simulink model "Vehicle_Model"  (R2018b)
settings: Solver=VariableStepAuto  StartTime=0.0  StopTime=60  FixedStep=0.00000000000000000000000000000000000000001  RelTol=1e-3
undefined symbols (not defined in the file or in its folder): Chassis8_Initial, Initial
(part 1 of 3)
settings Model: Creator=Foster  LastModifiedBy=Will

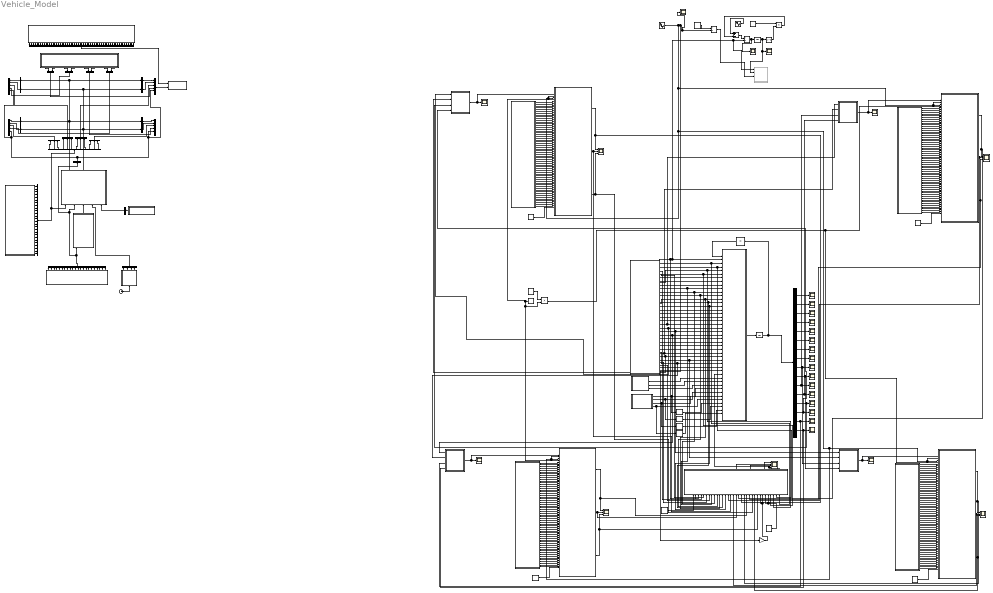
== system Vehicle_Model ==
  note: F=ma for Car in x
  note: Track Radius
  note: Track Curvature
  note: Tyre Model
  note: Rear Right
  note: Rear Left
  note: Front Right
  note: Front Left
  note: 8 DOF Chassis Ride Model
  note: Tyre Model
  note: Tyre Model
  note: Tyre Model
  Bus Creator : BusCreator  Inputs=22
  Bus Creator1 : BusCreator  Inputs=4
  Bus Creator{9..12} (4 alike) : BusCreator  Inputs=3
  Bus Creator{13..16} (4 alike) : BusCreator  Inputs=2
  Bus Creator{2..5} (4 alike) : BusCreator  Inputs=6
  Bus Creator6 : BusCreator  Inputs=59
  Bus Creator7 : BusCreator  Inputs=26
  Bus Creator8 : BusCreator  Inputs=1
  Bus Selector : BusSelector  OutputSignals=x_WFR
  Bus Selector1 : BusSelector  OutputSignals=x_WFL
  Bus Selector2 : BusSelector  OutputSignals=x_WRL
  Bus Selector3 : BusSelector  OutputSignals=x_WRR
  Bus Selector4 : BusSelector  OutputSignals=xdot_WFL
  Bus Selector5 : BusSelector  OutputSignals=xdot_WRL
  Bus Selector6 : BusSelector  OutputSignals=xdot_WFR
  Bus Selector7 : BusSelector  OutputSignals=xdot_WRR
  Bus Selector8 : BusSelector  OutputSignals=mu_scaling
  Bus Selector9 : BusSelector  OutputSignals=k_TRL,c_TRL,gamma_RL,k_TFL,c_TFL,gamma_FL,k_TFR,c_TFR,gamma_FR,k_TRR,c_TRR,gamma_RR
  Chassis Vertical 8DOF : Subsystem
  Clock : Clock
  Constant : Constant  Value=0.0175
  Constant{1..4} (4 alike) : Constant  Value=0.5
  Constant5 : Constant  Value=-1
  Constant6 : Constant
  Constant7 : Constant  Value=9.81
  Constant8 : Constant  Value=0
  Demux : Demux  Outputs=16
  Derivative{,1..3} (4 alike) : Derivative
  Divide : Product  Inputs=*/
  Divide1 : Product  Inputs=*/
  Drag Coefficient : Constant  Value=5
  Force_FL : Scope
  Force_FR : Scope
  Force_RL : Scope
  Force_RR : Scope
  Gain : Gain  Gain=50
  IC : InitialCondition  Value=Initial
  Integrator : Integrator
  Integrator1 : Integrator
  MATLAB Function : MATLAB Function  TreatAsAtomicUnit=on
  MATLAB Function1 : MATLAB Function  TreatAsAtomicUnit=on
  MATLAB Function10 : MATLAB Function  TreatAsAtomicUnit=on
  MATLAB Function11 : MATLAB Function  TreatAsAtomicUnit=on
  MATLAB Function12 : MATLAB Function  TreatAsAtomicUnit=on
  MATLAB Function13 : MATLAB Function  TreatAsAtomicUnit=on
  MATLAB Function14 : MATLAB Function  TreatAsAtomicUnit=on
  MATLAB Function15 : MATLAB Function  TreatAsAtomicUnit=on
  MATLAB Function16 : MATLAB Function  Commented=on  TreatAsAtomicUnit=on
  MATLAB Function17 : MATLAB Function  TreatAsAtomicUnit=on
  MATLAB Function18 : MATLAB Function  TreatAsAtomicUnit=on
  MATLAB Function19 : MATLAB Function  TreatAsAtomicUnit=on
  MATLAB Function2 : MATLAB Function  TreatAsAtomicUnit=on
  MATLAB Function20 : MATLAB Function  TreatAsAtomicUnit=on
  MATLAB Function21 : MATLAB Function  TreatAsAtomicUnit=on
  MATLAB Function22 : MATLAB Function  TreatAsAtomicUnit=on
  MATLAB Function23 : MATLAB Function  TreatAsAtomicUnit=on
  MATLAB Function3 : MATLAB Function  TreatAsAtomicUnit=on
  MATLAB Function4 : MATLAB Function  TreatAsAtomicUnit=on
  MATLAB Function5 : MATLAB Function  TreatAsAtomicUnit=on
  MATLAB Function6 : MATLAB Function  TreatAsAtomicUnit=on
  MATLAB Function7 : MATLAB Function  TreatAsAtomicUnit=on
  MATLAB Function8 : MATLAB Function  TreatAsAtomicUnit=on
  MATLAB Function9 : MATLAB Function  TreatAsAtomicUnit=on
  Minus : Sum  Inputs=+-
  Multiply : Product
  Multiply1 : Product
  Scope : Scope
  Scope{1..4} (4 alike) : Scope  NumInputPorts=3
  Scope5 : Scope  NumInputPorts=4
  Sine Wave : Sin  Amplitude=500  Bias=500  Frequency=0.5  SampleTime=0
  Square : Math  Operator=square  SaturateOnIntegerOverflow=on
  Subsystem : Subsystem
  Subsystem1 : Subsystem
  Track Curvature : Sin  Amplitude=0.01  Frequency=0.1  SampleTime=0
  a_x : Scope
  v_x : Scope
  x_WFL : Scope
  x_WFR : Scope
  x_WRL : Scope
  x_WRR : Scope
  x_thetaCF : Scope
  x_thetaCR : Scope
  xdot_WFL : Scope
  xdot_WFR : Scope
  xdot_WRL : Scope
  xdot_WRR : Scope
  xdot_thetaCF : Scope
  xdot_thetaCR : Scope
  y_thetaC : Scope
  ydot_thetaC : Scope
  z_C : Scope
  zdot_C : Scope
  wires:
  MATLAB Function1/1(m_C) -> MATLAB Function/2(m_C), MATLAB Function16/1(m_C), Divide1/2, MATLAB Function18/2(m_C)
  MATLAB Function1/4(m_WFR) -> MATLAB Function18/33(m_WFR), MATLAB Function/3(m_WFR)
  MATLAB Function1/5(m_WFL) -> MATLAB Function/4(m_WFL), MATLAB Function18/32(m_WFL)
  MATLAB Function1/6(m_WRR) -> MATLAB Function/5(m_WRR), MATLAB Function18/31(m_WRR)
  MATLAB Function1/7(m_WRL) -> MATLAB Function/6(m_WRL), MATLAB Function18/30(m_WRL)
  MATLAB Function1/8(I_Cy) -> MATLAB Function/7(I_Cy)
  MATLAB Function1/9(I_CFx) -> MATLAB Function/8(I_CFx)
  MATLAB Function1/10(I_CRx) -> MATLAB Function/9(I_CRx)
  MATLAB Function1/11(a) -> MATLAB Function/10(a), MATLAB Function18/8(a)
  MATLAB Function1/12(b) -> MATLAB Function18/9(b), MATLAB Function/11(b)
  MATLAB Function1/13(d_F) -> MATLAB Function18/10(d_F), MATLAB Function/12(d_F)
  MATLAB Function1/15(d_R) -> MATLAB Function/14(d_R), MATLAB Function18/12(d_R)
  MATLAB Function1/16(e_R) -> MATLAB Function/15(e_R), MATLAB Function18/13(e_R)
  MATLAB Function1/17(k_SFR) -> MATLAB Function/16(k_SFR)
  MATLAB Function1/18(k_SFL) -> MATLAB Function/17(k_SFL)
  MATLAB Function1/19(k_SRR) -> MATLAB Function/18(k_SRR)
  MATLAB Function1/20(k_SRL) -> MATLAB Function/19(k_SRL)
  MATLAB Function1/21(k_TFR) -> MATLAB Function4/1(k), MATLAB Function/20(k_TFR)
  MATLAB Function1/22(k_TFL) -> MATLAB Function7/1(k), MATLAB Function/21(k_TFL)
  MATLAB Function1/23(k_TRR) -> MATLAB Function6/1(k), MATLAB Function/22(k_TRR)
  MATLAB Function1/24(k_TRL) -> MATLAB Function5/1(k), MATLAB Function/23(k_TRL)
  MATLAB Function1/25(c_SFR) -> MATLAB Function/24(c_SFR)
  MATLAB Function1/26(c_SFL) -> MATLAB Function/25(c_SFL)
  MATLAB Function1/27(c_SRR) -> MATLAB Function/26(c_SRR)
  MATLAB Function1/28(c_SRL) -> MATLAB Function/27(c_SRL)
  MATLAB Function1/29(c_TFR) -> MATLAB Function4/2(c), MATLAB Function/28(c_TFR)
  MATLAB Function1/30(c_TFL) -> MATLAB Function7/2(c), MATLAB Function/29(c_TFL)
  MATLAB Function1/31(c_TRR) -> MATLAB Function6/2(c), MATLAB Function/30(c_TRR)
  MATLAB Function1/32(c_TRL) -> MATLAB Function5/2(c), MATLAB Function/31(c_TRL)
  MATLAB Function1/33(k_C) -> MATLAB Function/32(k_C)
  MATLAB Function1/34(c_C) -> MATLAB Function/33(c_C)
  MATLAB Function3/1(y_FR) -> Derivative/1, MATLAB Function/38(y_FR)
  MATLAB Function3/2(y_FL) -> Derivative1/1, MATLAB Function/39(y_FL)
  MATLAB Function3/3(y_RR) -> MATLAB Function/40(y_RR), Derivative2/1
  Derivative/1 -> MATLAB Function/42(ydot_FR)
  Derivative1/1 -> MATLAB Function/43(ydot_FL)
  Derivative2/1 -> MATLAB Function/44(ydot_RR)
  MATLAB Function/1(Z) -> Integrator/1
  Integrator/1 -> IC/1, Demux/1
  Demux/16 -> MATLAB Function5/4(xdot), xdot_WRL/1
  Demux/15 -> MATLAB Function5/3(x), x_WRL/1
  Demux/14 -> MATLAB Function7/4(xdot), xdot_WFL/1
  Demux/13 -> MATLAB Function7/3(x), x_WFL/1
  Demux/12 -> MATLAB Function4/4(xdot), xdot_WFR/1
  Demux/11 -> MATLAB Function4/3(x), x_WFR/1
  Demux/10 -> MATLAB Function6/4(xdot), xdot_WRR/1
  Demux/9 -> MATLAB Function6/3(x), x_WRR/1
  Demux/8 -> xdot_thetaCR/1
  Demux/7 -> x_thetaCR/1
  Demux/6 -> xdot_thetaCF/1
  Demux/5 -> x_thetaCF/1
  Demux/4 -> ydot_thetaC/1
  Demux/3 -> y_thetaC/1
  Demux/2 -> zdot_C/1
  Demux/1 -> z_C/1
  MATLAB Function7/1(F_z) -> MATLAB Function8/1(Fz), Force_FL/1
  MATLAB Function4/1(F_z) -> MATLAB Function14/1(Fz), Force_FR/1
  MATLAB Function6/1(F_z) -> MATLAB Function12/1(Fz), Force_RR/1
  MATLAB Function5/1(F_z) -> MATLAB Function10/1(Fz), Force_RL/1
  Derivative3/1 -> MATLAB Function/45(ydot_RL)
  MATLAB Function9/1(Fzo) -> MATLAB Function8/5(Fzo)
  MATLAB Function9/2(Ro) -> MATLAB Function8/6(Ro)
  MATLAB Function9/3(q_Bz1) -> MATLAB Function8/7(q_Bz1)
  MATLAB Function9/5(q_Bz3) -> MATLAB Function8/9(q_Bz3)
  MATLAB Function9/4(q_Bz2) -> MATLAB Function8/8(q_Bz2)
  MATLAB Function9/6(q_Bz4) -> MATLAB Function8/10(q_Bz4)
  MATLAB Function9/7(q_Bz5) -> MATLAB Function8/11(q_Bz5)
  MATLAB Function9/10(q_Cz1) -> MATLAB Function8/14(q_Cz1)
  MATLAB Function9/9(q_Bz10) -> MATLAB Function8/13(q_Bz10)
  MATLAB Function9/8(q_Bz9) -> MATLAB Function8/12(q_Bz9)
  MATLAB Function9/11(q_Dz1) -> MATLAB Function8/15(q_Dz1)
  MATLAB Function9/12(q_Dz2) -> MATLAB Function8/16(q_Dz2)
  MATLAB Function9/14(q_Dz4) -> MATLAB Function8/18(q_Dz4)
  MATLAB Function9/13(q_Dz3) -> MATLAB Function8/17(q_Dz3)
  MATLAB Function9/15(q_Dz6) -> MATLAB Function8/19(q_Dz6)
  MATLAB Function9/17(q_Dz8) -> MATLAB Function8/21(q_Dz8)
  MATLAB Function9/18(q_Dz9) -> MATLAB Function8/22(q_Dz9)
  MATLAB Function9/20(q_Ez2) -> MATLAB Function8/24(q_Ez2)
  MATLAB Function9/21(q_Ez3) -> MATLAB Function8/25(q_Ez3)
  MATLAB Function9/19(q_Ez1) -> MATLAB Function8/23(q_Ez1)
  MATLAB Function9/22(q_Ez4) -> MATLAB Function8/26(q_Ez4)
  MATLAB Function9/23(q_Ez5) -> MATLAB Function8/27(q_Ez5)
  MATLAB Function9/25(q_Hz2) -> MATLAB Function8/29(q_Hz2)
  MATLAB Function9/24(q_Hz1) -> MATLAB Function8/28(q_Hz1)
  MATLAB Function9/26(q_Hz3) -> MATLAB Function8/30(q_Hz3)
  MATLAB Function9/27(q_Hz4) -> MATLAB Function8/31(q_Hz4)
  MATLAB Function9/28(p_Cy1) -> MATLAB Function8/32(p_Cy1)
  MATLAB Function9/29(p_Dy1) -> MATLAB Function8/33(p_Dy1)
  MATLAB Function9/30(p_Dy2) -> MATLAB Function8/34(p_Dy2)
  MATLAB Function9/31(p_Dy3) -> MATLAB Function8/35(p_Dy3)
  MATLAB Function9/32(p_Ey1) -> MATLAB Function8/36(p_Ey1)
  MATLAB Function9/34(p_Ey3) -> MATLAB Function8/38(p_Ey3)
  MATLAB Function9/33(p_Ey2) -> MATLAB Function8/37(p_Ey2)
  MATLAB Function9/35(p_Ey4) -> MATLAB Function8/39(p_Ey4)
  MATLAB Function9/36(p_Ky1) -> MATLAB Function8/40(p_Ky1)
  MATLAB Function9/37(p_Ky2) -> MATLAB Function8/41(p_Ky2)
  MATLAB Function9/38(p_Ky3) -> MATLAB Function8/42(p_Ky3)
  MATLAB Function9/40(p_Hy2) -> MATLAB Function8/44(p_Hy2)
  MATLAB Function9/39(p_Hy1) -> MATLAB Function8/43(p_Hy1)
  MATLAB Function9/41(p_Hy3) -> MATLAB Function8/45(p_Hy3)
  MATLAB Function9/42(p_Vy1) -> MATLAB Function8/46(p_Vy1)
  MATLAB Function9/44(p_Vy3) -> MATLAB Function8/48(p_Vy3)
  MATLAB Function9/43(p_Vy2) -> MATLAB Function8/47(p_Vy2)
  MATLAB Function9/46(p_Cx1) -> MATLAB Function8/50(p_Cx1)
  MATLAB Function9/45(p_Vy4) -> MATLAB Function8/49(p_Vy4)
  MATLAB Function9/47(p_Dx1) -> MATLAB Function8/51(p_Dx1)
  MATLAB Function9/48(p_Dx2) -> MATLAB Function8/52(p_Dx2)
  MATLAB Function9/49(p_Ex1) -> MATLAB Function8/53(p_Ex1)
  MATLAB Function9/50(p_Ex2) -> MATLAB Function8/54(p_Ex2)
  MATLAB Function9/51(p_Ex3) -> MATLAB Function8/55(p_Ex3)
  MATLAB Function9/52(p_Ex4) -> MATLAB Function8/56(p_Ex4)
  MATLAB Function9/53(p_Kx1) -> MATLAB Function8/57(p_Kx1)
  MATLAB Function9/54(p_Kx2) -> MATLAB Function8/58(p_Kx2)
  MATLAB Function9/55(p_Kx3) -> MATLAB Function8/59(p_Kx3)
  MATLAB Function9/56(p_Hx1) -> MATLAB Function8/60(p_Hx1)
  MATLAB Function9/57(p_Hx2) -> MATLAB Function8/61(p_Hx2)
  MATLAB Function9/58(p_Vx1) -> MATLAB Function8/62(p_Vx1)
  MATLAB Function9/59(p_Vx2) -> MATLAB Function8/63(p_Vx2)
  Constant1/1 -> MATLAB Function8/64(car_mu_scaling)
  MATLAB Function9/16(q_Dz7) -> MATLAB Function8/20(q_Dz7)
  MATLAB Function8/1(Fxo) -> MATLAB Function18/19(F_xFL), Scope1/1
  MATLAB Function8/2(Fyo) -> MATLAB Function18/15(F_yFL), Scope1/2
  MATLAB Function8/3(Mzo) -> MATLAB Function18/23(M_zFL), Scope1/3
  MATLAB Function10/2(Fyo) -> MATLAB Function18/17(F_yRL), Scope2/2
  MATLAB Function11/56(p_Hx1) -> MATLAB Function10/60(p_Hx1)
  MATLAB Function11/40(p_Hy2) -> MATLAB Function10/44(p_Hy2)
  MATLAB Function11/9(q_Bz10) -> MATLAB Function10/13(q_Bz10)
  MATLAB Function11/26(q_Hz3) -> MATLAB Function10/30(q_Hz3)
  MATLAB Function11/52(p_Ex4) -> MATLAB Function10/56(p_Ex4)
  MATLAB Function11/35(p_Ey4) -> MATLAB Function10/39(p_Ey4)
  MATLAB Function11/5(q_Bz3) -> MATLAB Function10/9(q_Bz3)
  MATLAB Function11/7(q_Bz5) -> MATLAB Function10/11(q_Bz5)
  MATLAB Function11/21(q_Ez3) -> MATLAB Function10/25(q_Ez3)
  MATLAB Function11/38(p_Ky3) -> MATLAB Function10/42(p_Ky3)
  MATLAB Function11/14(q_Dz4) -> MATLAB Function10/18(q_Dz4)
  MATLAB Function11/51(p_Ex3) -> MATLAB Function10/55(p_Ex3)
  MATLAB Function11/45(p_Vy4) -> MATLAB Function10/49(p_Vy4)
  MATLAB Function11/18(q_Dz9) -> MATLAB Function10/22(q_Dz9)
  MATLAB Function11/37(p_Ky2) -> MATLAB Function10/41(p_Ky2)
  MATLAB Function11/39(p_Hy1) -> MATLAB Function10/43(p_Hy1)
  MATLAB Function11/55(p_Kx3) -> MATLAB Function10/59(p_Kx3)
  MATLAB Function11/59(p_Vx2) -> MATLAB Function10/63(p_Vx2)
  MATLAB Function11/4(q_Bz2) -> MATLAB Function10/8(q_Bz2)
  MATLAB Function11/24(q_Hz1) -> MATLAB Function10/28(q_Hz1)
  MATLAB Function11/15(q_Dz6) -> MATLAB Function10/19(q_Dz6)
  MATLAB Function11/41(p_Hy3) -> MATLAB Function10/45(p_Hy3)
  MATLAB Function10/3(Mzo) -> MATLAB Function18/25(M_zRL), Scope2/3
  MATLAB Function11/50(p_Ex2) -> MATLAB Function10/54(p_Ex2)
  MATLAB Function10/1(Fxo) -> MATLAB Function18/21(F_xRL), Scope2/1
  MATLAB Function11/49(p_Ex1) -> MATLAB Function10/53(p_Ex1)
  MATLAB Function11/46(p_Cx1) -> MATLAB Function10/50(p_Cx1)
  MATLAB Function11/58(p_Vx1) -> MATLAB Function10/62(p_Vx1)
  MATLAB Function11/47(p_Dx1) -> MATLAB Function10/51(p_Dx1)
  MATLAB Function11/48(p_Dx2) -> MATLAB Function10/52(p_Dx2)
  MATLAB Function11/2(Ro) -> MATLAB Function10/6(Ro)
  MATLAB Function11/57(p_Hx2) -> MATLAB Function10/61(p_Hx2)
  MATLAB Function11/54(p_Kx2) -> MATLAB Function10/58(p_Kx2)
  MATLAB Function11/16(q_Dz7) -> MATLAB Function10/20(q_Dz7)
  MATLAB Function11/53(p_Kx1) -> MATLAB Function10/57(p_Kx1)
  Constant2/1 -> MATLAB Function10/64(car_mu_scaling)
  MATLAB Function11/12(q_Dz2) -> MATLAB Function10/16(q_Dz2)
  MATLAB Function11/8(q_Bz9) -> MATLAB Function10/12(q_Bz9)
  MATLAB Function11/19(q_Ez1) -> MATLAB Function10/23(q_Ez1)
  MATLAB Function11/34(p_Ey3) -> MATLAB Function10/38(p_Ey3)
  MATLAB Function11/42(p_Vy1) -> MATLAB Function10/46(p_Vy1)
  MATLAB Function11/1(Fzo) -> MATLAB Function10/5(Fzo)
  MATLAB Function11/20(q_Ez2) -> MATLAB Function10/24(q_Ez2)
  MATLAB Function11/25(q_Hz2) -> MATLAB Function10/29(q_Hz2)
  MATLAB Function11/36(p_Ky1) -> MATLAB Function10/40(p_Ky1)
  MATLAB Function11/32(p_Ey1) -> MATLAB Function10/36(p_Ey1)
  MATLAB Function11/29(p_Dy1) -> MATLAB Function10/33(p_Dy1)
  MATLAB Function11/22(q_Ez4) -> MATLAB Function10/26(q_Ez4)
  MATLAB Function11/31(p_Dy3) -> MATLAB Function10/35(p_Dy3)
  MATLAB Function11/10(q_Cz1) -> MATLAB Function10/14(q_Cz1)
  MATLAB Function11/27(q_Hz4) -> MATLAB Function10/31(q_Hz4)
  MATLAB Function11/23(q_Ez5) -> MATLAB Function10/27(q_Ez5)
  MATLAB Function11/13(q_Dz3) -> MATLAB Function10/17(q_Dz3)
  MATLAB Function11/33(p_Ey2) -> MATLAB Function10/37(p_Ey2)
  MATLAB Function11/43(p_Vy2) -> MATLAB Function10/47(p_Vy2)
  MATLAB Function11/28(p_Cy1) -> MATLAB Function10/32(p_Cy1)
  MATLAB Function11/44(p_Vy3) -> MATLAB Function10/48(p_Vy3)
  MATLAB Function11/3(q_Bz1) -> MATLAB Function10/7(q_Bz1)
  MATLAB Function11/30(p_Dy2) -> MATLAB Function10/34(p_Dy2)
  MATLAB Function11/17(q_Dz8) -> MATLAB Function10/21(q_Dz8)
  MATLAB Function11/6(q_Bz4) -> MATLAB Function10/10(q_Bz4)
  MATLAB Function11/11(q_Dz1) -> MATLAB Function10/15(q_Dz1)
  MATLAB Function13/27(q_Hz4) -> MATLAB Function12/31(q_Hz4)
  MATLAB Function13/18(q_Dz9) -> MATLAB Function12/22(q_Dz9)
  MATLAB Function13/9(q_Bz10) -> MATLAB Function12/13(q_Bz10)
  MATLAB Function13/42(p_Vy1) -> MATLAB Function12/46(p_Vy1)
  MATLAB Function13/45(p_Vy4) -> MATLAB Function12/49(p_Vy4)
  MATLAB Function13/30(p_Dy2) -> MATLAB Function12/34(p_Dy2)
  MATLAB Function13/33(p_Ey2) -> MATLAB Function12/37(p_Ey2)
  MATLAB Function13/37(p_Ky2) -> MATLAB Function12/41(p_Ky2)
  MATLAB Function13/7(q_Bz5) -> MATLAB Function12/11(q_Bz5)
  MATLAB Function13/20(q_Ez2) -> MATLAB Function12/24(q_Ez2)
  MATLAB Function13/52(p_Ex4) -> MATLAB Function12/56(p_Ex4)
  MATLAB Function13/28(p_Cy1) -> MATLAB Function12/32(p_Cy1)
  MATLAB Function13/43(p_Vy2) -> MATLAB Function12/47(p_Vy2)
  MATLAB Function13/22(q_Ez4) -> MATLAB Function12/26(q_Ez4)
  MATLAB Function13/21(q_Ez3) -> MATLAB Function12/25(q_Ez3)
  MATLAB Function13/44(p_Vy3) -> MATLAB Function12/48(p_Vy3)
  MATLAB Function13/31(p_Dy3) -> MATLAB Function12/35(p_Dy3)
  MATLAB Function13/55(p_Kx3) -> MATLAB Function12/59(p_Kx3)
  MATLAB Function13/39(p_Hy1) -> MATLAB Function12/43(p_Hy1)
  MATLAB Function13/11(q_Dz1) -> MATLAB Function12/15(q_Dz1)
  MATLAB Function12/2(Fyo) -> MATLAB Function18/16(F_yRR), Scope3/2
  MATLAB Function13/56(p_Hx1) -> MATLAB Function12/60(p_Hx1)
  MATLAB Function13/5(q_Bz3) -> MATLAB Function12/9(q_Bz3)
  MATLAB Function13/14(q_Dz4) -> MATLAB Function12/18(q_Dz4)
  MATLAB Function13/35(p_Ey4) -> MATLAB Function12/39(p_Ey4)
  MATLAB Function13/13(q_Dz3) -> MATLAB Function12/17(q_Dz3)
  MATLAB Function13/40(p_Hy2) -> MATLAB Function12/44(p_Hy2)
  MATLAB Function13/46(p_Cx1) -> MATLAB Function12/50(p_Cx1)
  MATLAB Function13/19(q_Ez1) -> MATLAB Function12/23(q_Ez1)
  MATLAB Function13/36(p_Ky1) -> MATLAB Function12/40(p_Ky1)
  MATLAB Function13/38(p_Ky3) -> MATLAB Function12/42(p_Ky3)
  MATLAB Function13/59(p_Vx2) -> MATLAB Function12/63(p_Vx2)
  MATLAB Function13/4(q_Bz2) -> MATLAB Function12/8(q_Bz2)
  MATLAB Function13/32(p_Ey1) -> MATLAB Function12/36(p_Ey1)
  MATLAB Function13/12(q_Dz2) -> MATLAB Function12/16(q_Dz2)
  MATLAB Function13/6(q_Bz4) -> MATLAB Function12/10(q_Bz4)
  MATLAB Function13/3(q_Bz1) -> MATLAB Function12/7(q_Bz1)
  MATLAB Function13/15(q_Dz6) -> MATLAB Function12/19(q_Dz6)
  MATLAB Function13/8(q_Bz9) -> MATLAB Function12/12(q_Bz9)
  Constant3/1 -> MATLAB Function12/64(car_mu_scaling)
  MATLAB Function13/10(q_Cz1) -> MATLAB Function12/14(q_Cz1)
  MATLAB Function13/26(q_Hz3) -> MATLAB Function12/30(q_Hz3)
  MATLAB Function12/1(Fxo) -> MATLAB Function18/20(F_xRR), Scope3/1
  MATLAB Function13/1(Fzo) -> MATLAB Function12/5(Fzo)
  MATLAB Function13/34(p_Ey3) -> MATLAB Function12/38(p_Ey3)
  MATLAB Function13/41(p_Hy3) -> MATLAB Function12/45(p_Hy3)
  MATLAB Function13/23(q_Ez5) -> MATLAB Function12/27(q_Ez5)
  MATLAB Function13/51(p_Ex3) -> MATLAB Function12/55(p_Ex3)
  MATLAB Function13/29(p_Dy1) -> MATLAB Function12/33(p_Dy1)
  MATLAB Function13/17(q_Dz8) -> MATLAB Function12/21(q_Dz8)
  MATLAB Function13/25(q_Hz2) -> MATLAB Function12/29(q_Hz2)
  MATLAB Function13/16(q_Dz7) -> MATLAB Function12/20(q_Dz7)
  MATLAB Function13/2(Ro) -> MATLAB Function12/6(Ro)
  MATLAB Function13/48(p_Dx2) -> MATLAB Function12/52(p_Dx2)
  MATLAB Function13/47(p_Dx1) -> MATLAB Function12/51(p_Dx1)
  MATLAB Function13/53(p_Kx1) -> MATLAB Function12/57(p_Kx1)
  MATLAB Function13/54(p_Kx2) -> MATLAB Function12/58(p_Kx2)
  MATLAB Function13/49(p_Ex1) -> MATLAB Function12/53(p_Ex1)
  MATLAB Function13/24(q_Hz1) -> MATLAB Function12/28(q_Hz1)
  MATLAB Function13/57(p_Hx2) -> MATLAB Function12/61(p_Hx2)
  MATLAB Function12/3(Mzo) -> Scope3/3, MATLAB Function18/24(M_zRR)
  MATLAB Function13/58(p_Vx1) -> MATLAB Function12/62(p_Vx1)
  MATLAB Function13/50(p_Ex2) -> MATLAB Function12/54(p_Ex2)
  MATLAB Function15/27(q_Hz4) -> MATLAB Function14/31(q_Hz4)
  MATLAB Function15/18(q_Dz9) -> MATLAB Function14/22(q_Dz9)
  MATLAB Function15/9(q_Bz10) -> MATLAB Function14/13(q_Bz10)
  MATLAB Function15/42(p_Vy1) -> MATLAB Function14/46(p_Vy1)
  MATLAB Function15/45(p_Vy4) -> MATLAB Function14/49(p_Vy4)
  MATLAB Function15/30(p_Dy2) -> MATLAB Function14/34(p_Dy2)
  MATLAB Function15/33(p_Ey2) -> MATLAB Function14/37(p_Ey2)
  MATLAB Function15/37(p_Ky2) -> MATLAB Function14/41(p_Ky2)
  MATLAB Function15/7(q_Bz5) -> MATLAB Function14/11(q_Bz5)
  MATLAB Function15/20(q_Ez2) -> MATLAB Function14/24(q_Ez2)
  MATLAB Function15/52(p_Ex4) -> MATLAB Function14/56(p_Ex4)
  MATLAB Function15/28(p_Cy1) -> MATLAB Function14/32(p_Cy1)
  MATLAB Function15/43(p_Vy2) -> MATLAB Function14/47(p_Vy2)
  MATLAB Function15/22(q_Ez4) -> MATLAB Function14/26(q_Ez4)
  MATLAB Function15/21(q_Ez3) -> MATLAB Function14/25(q_Ez3)
  MATLAB Function15/44(p_Vy3) -> MATLAB Function14/48(p_Vy3)
  MATLAB Function15/31(p_Dy3) -> MATLAB Function14/35(p_Dy3)
  MATLAB Function15/55(p_Kx3) -> MATLAB Function14/59(p_Kx3)
  MATLAB Function15/39(p_Hy1) -> MATLAB Function14/43(p_Hy1)
  MATLAB Function15/11(q_Dz1) -> MATLAB Function14/15(q_Dz1)
  MATLAB Function14/2(Fyo) -> MATLAB Function18/14(F_yFR), Scope4/2
  MATLAB Function15/56(p_Hx1) -> MATLAB Function14/60(p_Hx1)
  MATLAB Function15/5(q_Bz3) -> MATLAB Function14/9(q_Bz3)
  MATLAB Function15/14(q_Dz4) -> MATLAB Function14/18(q_Dz4)
  MATLAB Function15/35(p_Ey4) -> MATLAB Function14/39(p_Ey4)
  MATLAB Function15/13(q_Dz3) -> MATLAB Function14/17(q_Dz3)
  MATLAB Function15/40(p_Hy2) -> MATLAB Function14/44(p_Hy2)
  MATLAB Function15/46(p_Cx1) -> MATLAB Function14/50(p_Cx1)
  MATLAB Function15/19(q_Ez1) -> MATLAB Function14/23(q_Ez1)
  MATLAB Function15/36(p_Ky1) -> MATLAB Function14/40(p_Ky1)
  MATLAB Function15/38(p_Ky3) -> MATLAB Function14/42(p_Ky3)
  MATLAB Function15/59(p_Vx2) -> MATLAB Function14/63(p_Vx2)
  MATLAB Function15/4(q_Bz2) -> MATLAB Function14/8(q_Bz2)
  MATLAB Function15/32(p_Ey1) -> MATLAB Function14/36(p_Ey1)
  MATLAB Function15/12(q_Dz2) -> MATLAB Function14/16(q_Dz2)
  MATLAB Function15/6(q_Bz4) -> MATLAB Function14/10(q_Bz4)
  MATLAB Function15/3(q_Bz1) -> MATLAB Function14/7(q_Bz1)
  MATLAB Function15/15(q_Dz6) -> MATLAB Function14/19(q_Dz6)
  MATLAB Function15/8(q_Bz9) -> MATLAB Function14/12(q_Bz9)
  Constant4/1 -> MATLAB Function14/64(car_mu_scaling)
  MATLAB Function15/10(q_Cz1) -> MATLAB Function14/14(q_Cz1)
  MATLAB Function15/26(q_Hz3) -> MATLAB Function14/30(q_Hz3)
  MATLAB Function14/1(Fxo) -> MATLAB Function18/18(F_xFR), Scope4/1
  MATLAB Function15/1(Fzo) -> MATLAB Function14/5(Fzo)
  MATLAB Function15/34(p_Ey3) -> MATLAB Function14/38(p_Ey3)
  MATLAB Function15/41(p_Hy3) -> MATLAB Function14/45(p_Hy3)
  MATLAB Function15/23(q_Ez5) -> MATLAB Function14/27(q_Ez5)
  MATLAB Function15/51(p_Ex3) -> MATLAB Function14/55(p_Ex3)
  MATLAB Function15/29(p_Dy1) -> MATLAB Function14/33(p_Dy1)
  MATLAB Function15/17(q_Dz8) -> MATLAB Function14/21(q_Dz8)
  MATLAB Function15/25(q_Hz2) -> MATLAB Function14/29(q_Hz2)
  MATLAB Function15/16(q_Dz7) -> MATLAB Function14/20(q_Dz7)
  MATLAB Function15/2(Ro) -> MATLAB Function14/6(Ro)
  MATLAB Function15/48(p_Dx2) -> MATLAB Function14/52(p_Dx2)
  MATLAB Function15/47(p_Dx1) -> MATLAB Function14/51(p_Dx1)
  MATLAB Function15/53(p_Kx1) -> MATLAB Function14/57(p_Kx1)
  MATLAB Function15/54(p_Kx2) -> MATLAB Function14/58(p_Kx2)
  MATLAB Function15/49(p_Ex1) -> MATLAB Function14/53(p_Ex1)
  MATLAB Function15/24(q_Hz1) -> MATLAB Function14/28(q_Hz1)
  MATLAB Function15/57(p_Hx2) -> MATLAB Function14/61(p_Hx2)
  MATLAB Function14/3(Mzo) -> MATLAB Function18/22(M_zFR), Scope4/3
  MATLAB Function15/58(p_Vx1) -> MATLAB Function14/62(p_Vx1)
  MATLAB Function15/50(p_Ex2) -> MATLAB Function14/54(p_Ex2)
  MATLAB Function3/4(y_RL) -> Derivative3/1, MATLAB Function/41(y_RL)
  Constant/1 -> Multiply/2, MATLAB Function10/4(gam), MATLAB Function8/4(gam)
  Constant5/1 -> Multiply/1
  Multiply/1 -> MATLAB Function12/4(gam), MATLAB Function14/4(gam)
  Constant6/1 -> Divide/1
  Divide1/1 -> a_x/1, Integrator1/1
  Integrator1/1 -> MATLAB Function16/2("v_x "), v_x/1, Square/1
  Square/1 -> Multiply1/2
  Drag Coefficient/1 -> Multiply1/1
  Sine Wave/1 -> Minus/1
  Minus/1 -> Divide1/1
  Divide/1 -> MATLAB Function16/3(r)
  Multiply1/1 -> Minus/2
  Track Curvature/1 -> Gain/1, Scope/1, Divide/2, MATLAB Function14/2(kappa), MATLAB Function14/3(alpha), MATLAB Function10/2(kappa), MATLAB Function10/3(alpha), MATLAB Function12/2(kappa), MATLAB Function12/3(alpha), MATLAB Function8/2(kappa), MATLAB Function8/3(alpha)
  MATLAB Function1/3(m_CR) -> MATLAB Function18/5(m_CR)
  MATLAB Function1/2(m_CF) -> MATLAB Function18/4(m_CF)
  Constant7/1 -> MATLAB Function18/1(g)
  MATLAB Function1/35(h_C) -> MATLAB Function18/3(h_C)
  MATLAB Function1/36(h_CF) -> MATLAB Function18/6(h_CF)
  MATLAB Function1/37(h_CR) -> MATLAB Function18/7(h_CR)
  MATLAB Function1/14(e_F) -> MATLAB Function18/11(e_F), MATLAB Function/13(e_F)
  Gain/1 -> MATLAB Function18/27(S_FL), MATLAB Function18/26(S_FR)
  Constant8/1 -> MATLAB Function18/29(S_RL), MATLAB Function18/28(S_RR)
  IC/1 -> MATLAB Function/1(z)
  MATLAB Function18/7(F_z) -> MATLAB Function/34(F_z), Scope5/4
  MATLAB Function2/3(M_xF) -> MATLAB Function/36(M_xF)
  MATLAB Function2/4(M_xR) -> MATLAB Function/37(M_xR)
  MATLAB Function18/6(M_xR) -> Scope5/1
  MATLAB Function18/5(M_xF) -> Scope5/3
  MATLAB Function18/4(M_y) -> Scope5/2
  MATLAB Function2/2(M_y) -> MATLAB Function/35(M_y)
  MATLAB Function17/1(m_C) -> Bus Creator/1
  MATLAB Function17/2(m_CF) -> Bus Creator/2
  MATLAB Function17/3(m_CR) -> Bus Creator/3
  MATLAB Function17/4(m_WFR) -> Bus Creator/4
  MATLAB Function17/5(m_WFL) -> Bus Creator/5
  MATLAB Function17/6(m_WRR) -> Bus Creator/6
  MATLAB Function17/7(m_WRL) -> Bus Creator/7
  MATLAB Function17/8(I_Cy) -> Bus Creator/8
  MATLAB Function17/9(I_CFx) -> Bus Creator/9
  MATLAB Function17/10(I_CRx) -> Bus Creator/10
  MATLAB Function17/11(a) -> Bus Creator/11
  MATLAB Function17/12(b) -> Bus Creator/12
  MATLAB Function17/13(d_F) -> Bus Creator/13
  MATLAB Function17/14(e_F) -> Bus Creator/14
  MATLAB Function17/15(d_R) -> Bus Creator/15
  MATLAB Function17/16(e_R) -> Bus Creator/16
  MATLAB Function17/17(k_C) -> Bus Creator/17
  MATLAB Function17/18(c_C) -> Bus Creator/18
  MATLAB Function17/19(h_C) -> Bus Creator/19
  MATLAB Function17/20(h_CF) -> Bus Creator/20
  MATLAB Function17/21(h_CR) -> Bus Creator/21
  Bus Creator/1 -> Bus Selector8/1, Chassis Vertical 8DOF/2(Car Parameters), Subsystem/1(Car Parameters)
  MATLAB Function19/1(y_FR) -> Bus Creator1/1
  MATLAB Function19/2(y_FL) -> Bus Creator1/2
  MATLAB Function19/3(y_RR) -> Bus Creator1/3
  MATLAB Function19/4(y_RL) -> Bus Creator1/4
  Bus Creator1/1 -> Chassis Vertical 8DOF/4(Base Excitation)
  Clock/1 -> MATLAB Function19/1(t)
  Subsystem/1(Chassis Forces) -> Chassis Vertical 8DOF/3(Chassis Forces)
  Chassis Vertical 8DOF/1(Vertical Displacements) -> Bus Selector1/1, Bus Selector/1, Bus Selector3/1, Bus Selector2/1
  Chassis Vertical 8DOF/2(Vertical Velocities) -> Bus Selector6/1, Bus Selector4/1, Bus Selector7/1, Bus Selector5/1
  Bus Selector2/1 -> Bus Creator3/1  "<x_WRL>"
  Bus Selector5/1 -> Bus Creator3/2  "<xdot_WRL>"
  Bus Selector8/1 -> Bus Creator5/5, Bus Creator4/5, Bus Creator3/5, Bus Creator2/5  "<mu_scaling>"
  Bus Selector1/1 -> Bus Creator2/1  "<x_WFL>"
  Bus Selector4/1 -> Bus Creator2/2  "<xdot_WFL>"
  Bus Selector/1 -> Bus Creator4/1  "<x_WFR>"
  Bus Selector6/1 -> Bus Creator4/2  "<xdot_WFR>"
  Bus Selector3/1 -> Bus Creator5/1  "<x_WRR>"
  Bus Selector7/1 -> Bus Creator5/2  "<xdot_WRR>"
  MATLAB Function20/1(Fzo) -> Bus Creator6/1
  MATLAB Function20/2(Ro) -> Bus Creator6/2
  MATLAB Function20/3(q_Bz1) -> Bus Creator6/3
  MATLAB Function20/4(q_Bz2) -> Bus Creator6/4
  MATLAB Function20/5(q_Bz3) -> Bus Creator6/5
  MATLAB Function20/6(q_Bz4) -> Bus Creator6/6
  MATLAB Function20/7(q_Bz5) -> Bus Creator6/7
  MATLAB Function20/8(q_Bz9) -> Bus Creator6/8
  MATLAB Function20/9(q_Bz10) -> Bus Creator6/9
  MATLAB Function20/10(q_Cz1) -> Bus Creator6/10
  MATLAB Function20/11(q_Dz1) -> Bus Creator6/11
  MATLAB Function20/12(q_Dz2) -> Bus Creator6/12
  MATLAB Function20/13(q_Dz3) -> Bus Creator6/13
  MATLAB Function20/14(q_Dz4) -> Bus Creator6/14
  MATLAB Function20/15(q_Dz6) -> Bus Creator6/15
  MATLAB Function20/16(q_Dz7) -> Bus Creator6/16
  MATLAB Function20/17(q_Dz8) -> Bus Creator6/17
  MATLAB Function20/18(q_Dz9) -> Bus Creator6/18
  MATLAB Function20/19(q_Ez1) -> Bus Creator6/19
  MATLAB Function20/20(q_Ez2) -> Bus Creator6/20
  MATLAB Function20/21(q_Ez3) -> Bus Creator6/21
  MATLAB Function20/22(q_Ez4) -> Bus Creator6/22
  MATLAB Function20/23(q_Ez5) -> Bus Creator6/23
  MATLAB Function20/24(q_Hz1) -> Bus Creator6/24
  MATLAB Function20/25(q_Hz2) -> Bus Creator6/25
  MATLAB Function20/26(q_Hz3) -> Bus Creator6/26
  MATLAB Function20/27(q_Hz4) -> Bus Creator6/27
  MATLAB Function20/28(p_Cy1) -> Bus Creator6/28
  MATLAB Function20/29(p_Dy1) -> Bus Creator6/29
  MATLAB Function20/30(p_Dy2) -> Bus Creator6/30
  MATLAB Function20/31(p_Dy3) -> Bus Creator6/31
  MATLAB Function20/32(p_Ey1) -> Bus Creator6/32
  MATLAB Function20/33(p_Ey2) -> Bus Creator6/33
  MATLAB Function20/34(p_Ey3) -> Bus Creator6/34
  MATLAB Function20/35(p_Ey4) -> Bus Creator6/35
  MATLAB Function20/36(p_Ky1) -> Bus Creator6/36
  MATLAB Function20/37(p_Ky2) -> Bus Creator6/37
  MATLAB Function20/38(p_Ky3) -> Bus Creator6/38
  MATLAB Function20/39(p_Hy1) -> Bus Creator6/39
  MATLAB Function20/40(p_Hy2) -> Bus Creator6/40
  MATLAB Function20/41(p_Hy3) -> Bus Creator6/41
  MATLAB Function20/42(p_Vy1) -> Bus Creator6/42
  MATLAB Function20/43(p_Vy2) -> Bus Creator6/43
  MATLAB Function20/44(p_Vy3) -> Bus Creator6/44
  MATLAB Function20/45(p_Vy4) -> Bus Creator6/45
  MATLAB Function20/46(p_Cx1) -> Bus Creator6/46
  MATLAB Function20/47(p_Dx1) -> Bus Creator6/47
  MATLAB Function20/48(p_Dx2) -> Bus Creator6/48
  MATLAB Function20/49(p_Ex1) -> Bus Creator6/49
  MATLAB Function20/50(p_Ex2) -> Bus Creator6/50
  MATLAB Function20/51(p_Ex3) -> Bus Creator6/51
  MATLAB Function20/52(p_Ex4) -> Bus Creator6/52
  MATLAB Function20/53(p_Kx1) -> Bus Creator6/53
  MATLAB Function20/54(p_Kx2) -> Bus Creator6/54
  MATLAB Function20/55(p_Kx3) -> Bus Creator6/55
  MATLAB Function20/56(p_Hx1) -> Bus Creator6/56
  MATLAB Function20/57(p_Hx2) -> Bus Creator6/57
  MATLAB Function20/58(p_Vx1) -> Bus Creator6/58
  MATLAB Function20/59(p_Vx2) -> Bus Creator6/59
  Bus Creator4/1 -> Subsystem1/2(Tyre Dynamics)
  Bus Creator6/1 -> Subsystem1/1(Tyre Coefficients)
  MATLAB Function21/1(k_SFR) -> Bus Creator7/1
  MATLAB Function21/2(k_SFL) -> Bus Creator7/2
  MATLAB Function21/3(k_SRR) -> Bus Creator7/3
  MATLAB Function21/4(k_SRL) -> Bus Creator7/4
  MATLAB Function21/5(c_SFR) -> Bus Creator7/5
  MATLAB Function21/6(c_SFL) -> Bus Creator7/6
  MATLAB Function21/7(c_SRR) -> Bus Creator7/7
  MATLAB Function21/8(c_SRL) -> Bus Creator7/8
  MATLAB Function21/9(k_TFR) -> Bus Creator7/9
  MATLAB Function21/10(k_TFL) -> Bus Creator7/10
  MATLAB Function21/11(k_TRR) -> Bus Creator7/11
  MATLAB Function21/12(k_TRL) -> Bus Creator7/12
  MATLAB Function21/13(c_TFR) -> Bus Creator7/13
  MATLAB Function21/14(c_TFL) -> Bus Creator7/14
  MATLAB Function21/15(c_TRR) -> Bus Creator7/15
  MATLAB Function21/16(c_TRL) -> Bus Creator7/16
  MATLAB Function21/17(k_RF) -> Bus Creator7/17
  MATLAB Function21/18(k_RR) -> Bus Creator7/18
  MATLAB Function21/19(k_FRIC) -> Bus Creator7/19
  MATLAB Function21/20(c_RF) -> Bus Creator7/20
  MATLAB Function21/21(c_RR) -> Bus Creator7/21
  MATLAB Function21/22(c_FRIC) -> Bus Creator7/22
  Bus Creator7/1 -> Bus Selector9/1, Chassis Vertical 8DOF/1(Suspension Parameters)
  MATLAB Function22/1(g) -> Bus Creator8/1
  Bus Creator8/1 -> Chassis Vertical 8DOF/5(Environment Parameters)
  MATLAB Function17/22(mu_scaling) -> Bus Creator/22
  MATLAB Function21/23(gamma_FR) -> Bus Creator7/23
  MATLAB Function21/24(gamma_FL) -> Bus Creator7/24
  MATLAB Function21/25(gamma_RR) -> Bus Creator7/25
  MATLAB Function21/26(gamma_RL) -> Bus Creator7/26
  Bus Selector9/1 -> Bus Creator9/1  "<k_TRL>"
  Bus Selector9/2 -> Bus Creator9/2  "<c_TRL>"
  Bus Selector9/3 -> Bus Creator9/3  "<gamma_RL>"
  Bus Creator9/1 -> Bus Creator3/3
  Bus Selector9/4 -> Bus Creator10/1  "<k_TFL>"
  Bus Selector9/5 -> Bus Creator10/2  "<c_TFL>"
  Bus Selector9/6 -> Bus Creator10/3  "<gamma_FL>"
  Bus Creator10/1 -> Bus Creator2/3
  Bus Selector9/11 -> Bus Creator12/2  "<c_TRR>"
  Bus Selector9/10 -> Bus Creator12/1  "<k_TRR>"
  Bus Selector9/12 -> Bus Creator12/3  "<gamma_RR>"
  Bus Selector9/8 -> Bus Creator11/2  "<c_TFR>"
  Bus Selector9/7 -> Bus Creator11/1  "<k_TFR>"
  Bus Selector9/9 -> Bus Creator11/3  "<gamma_FR>"
  Bus Creator11/1 -> Bus Creator4/3
  Bus Creator12/1 -> Bus Creator5/3
  MATLAB Function23/1(ratio_FR) -> Bus Creator13/1
  MATLAB Function23/2(angle_FR) -> Bus Creator13/2
  MATLAB Function23/3(ratio_FL) -> Bus Creator14/1
  MATLAB Function23/4(angle_FL) -> Bus Creator14/2
  MATLAB Function23/5(ratio_RR) -> Bus Creator15/1
  MATLAB Function23/6(angle_RR) -> Bus Creator15/2
  MATLAB Function23/7(ratio_RL) -> Bus Creator16/1
  MATLAB Function23/8(angle_RL) -> Bus Creator16/2
  Bus Creator13/1 -> Bus Creator4/4
  Bus Creator14/1 -> Bus Creator2/4
  Bus Creator15/1 -> Bus Creator5/4
  Bus Creator16/1 -> Bus Creator3/4

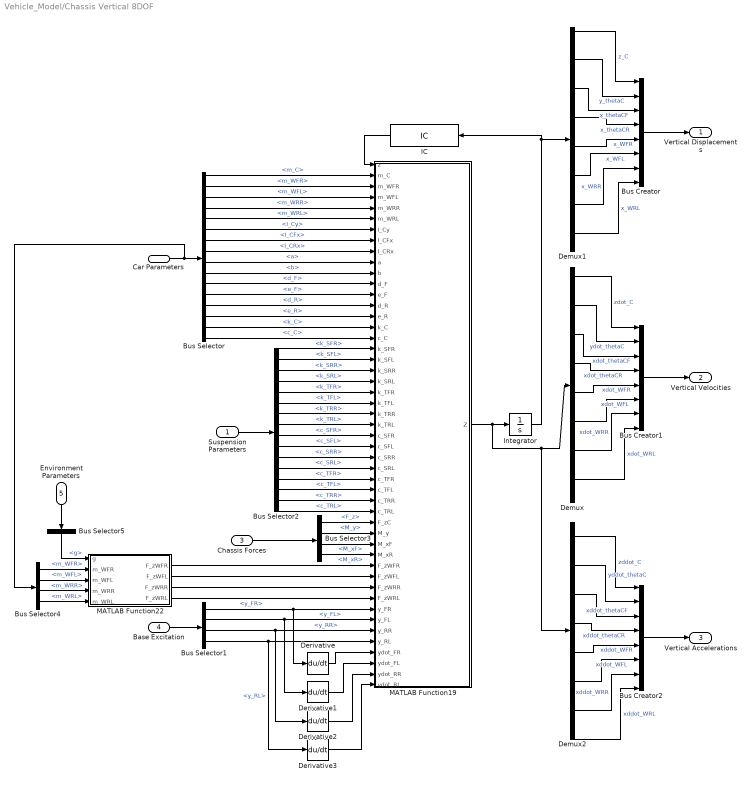
== system Vehicle_Model/Chassis Vertical 8DOF ==
  Suspension Parameters : Inport
  Car Parameters : Inport  Port=2
  Chassis Forces : Inport  Port=3
  Base Excitation : Inport  Port=4
  Environment Parameters : Inport  Port=5
  Bus Creator : BusCreator  Inputs=8
  Bus Creator1 : BusCreator  Inputs=8
  Bus Creator2 : BusCreator  Inputs=8
  Bus Selector : BusSelector  OutputSignals=m_C,m_WFR,m_WFL,m_WRR,m_WRL,I_Cy,I_CFx,I_CRx,a,b,d_F,e_F,d_R,e_R,k_C,c_C
  Bus Selector1 : BusSelector  OutputSignals=y_FR,y_FL,y_RR,y_RL
  Bus Selector2 : BusSelector  OutputSignals=k_SFR,k_SFL,k_SRR,k_SRL,k_TFR,k_TFL,k_TRR,k_TRL,c_SFR,c_SFL,c_SRR,c_SRL,c_TFR,c_TFL,c_TRR,c_TRL
  Bus Selector3 : BusSelector  OutputSignals=F_z,M_y,M_xF,M_xR
  Bus Selector4 : BusSelector  OutputSignals=m_WFR,m_WFL,m_WRR,m_WRL
  Bus Selector5 : BusSelector  OutputSignals=g
  Demux : Demux  Outputs=16
  Demux1 : Demux  Outputs=16
  Demux2 : Demux  Outputs=16
  Derivative{,1..3} (4 alike) : Derivative
  IC : InitialCondition  Value=Chassis8_Initial
  Integrator : Integrator
  MATLAB Function19 : MATLAB Function  TreatAsAtomicUnit=on
  MATLAB Function22 : MATLAB Function  TreatAsAtomicUnit=on
  Vertical Displacements : Outport
  Vertical Velocities : Outport  Port=2
  Vertical Accelerations : Outport  Port=3
  wires:
  Car Parameters/1 -> Bus Selector4/1, Bus Selector/1
  Bus Selector/1 -> MATLAB Function19/2(m_C)  "<m_C>"
  Bus Selector/2 -> MATLAB Function19/3(m_WFR)  "<m_WFR>"
  Bus Selector/3 -> MATLAB Function19/4(m_WFL)  "<m_WFL>"
  Bus Selector/4 -> MATLAB Function19/5(m_WRR)  "<m_WRR>"
  Bus Selector/5 -> MATLAB Function19/6(m_WRL)  "<m_WRL>"
  Bus Selector/6 -> MATLAB Function19/7(I_Cy)  "<I_Cy>"
  Bus Selector/7 -> MATLAB Function19/8(I_CFx)  "<I_CFx>"
  Bus Selector/8 -> MATLAB Function19/9(I_CRx)  "<I_CRx>"
  Bus Selector/9 -> MATLAB Function19/10(a)  "<a>"
  Bus Selector/10 -> MATLAB Function19/11(b)  "<b>"
  Bus Selector/11 -> MATLAB Function19/12(d_F)  "<d_F>"
  Bus Selector/12 -> MATLAB Function19/13(e_F)  "<e_F>"
  Bus Selector/13 -> MATLAB Function19/14(d_R)  "<d_R>"
  Bus Selector/14 -> MATLAB Function19/15(e_R)  "<e_R>"
  Bus Selector/15 -> MATLAB Function19/16(k_C)  "<k_C>"
  Bus Selector/16 -> MATLAB Function19/17(c_C)  "<c_C>"
  IC/1 -> MATLAB Function19/1(z)
  MATLAB Function19/1(Z) -> Demux2/1, Demux/1, Integrator/1
  Integrator/1 -> Demux1/1, IC/1
  Demux1/1 -> Bus Creator/1  "z_C"
  Demux1/3 -> Bus Creator/2  "y_thetaC"
  Demux1/5 -> Bus Creator/3  "x_thetaCF"
  Demux1/7 -> Bus Creator/4  "x_thetaCR"
  Demux1/9 -> Bus Creator/5  "x_WFR"
  Demux1/11 -> Bus Creator/6  "x_WFL"
  Demux1/13 -> Bus Creator/7  "x_WRR"
  Demux1/15 -> Bus Creator/8  "x_WRL"
  Bus Creator/1 -> Vertical Displacements/1
  Bus Creator1/1 -> Vertical Velocities/1
  Bus Creator2/1 -> Vertical Accelerations/1
  Demux/1 -> Bus Creator1/1  "zdot_C"
  Demux/3 -> Bus Creator1/2  "ydot_thetaC"
  Demux/5 -> Bus Creator1/3  "xdot_thetaCF"
  Demux/7 -> Bus Creator1/4  "xdot_thetaCR"
  Demux/9 -> Bus Creator1/5  "xdot_WFR"
  Demux/11 -> Bus Creator1/6  "xdot_WFL"
  Demux/13 -> Bus Creator1/7  "xdot_WRR"
  Demux/15 -> Bus Creator1/8  "xdot_WRL"
  Demux2/2 -> Bus Creator2/1  "zddot_C"
  Demux2/4 -> Bus Creator2/2  "yddot_thetaC"
  Demux2/6 -> Bus Creator2/3  "xddot_thetaCF"
  Demux2/8 -> Bus Creator2/4  "xddot_thetaCR"
  Demux2/10 -> Bus Creator2/5  "xddot_WFR"
  Demux2/12 -> Bus Creator2/6  "xddot_WFL"
  Demux2/14 -> Bus Creator2/7  "xddot_WRR"
  Demux2/16 -> Bus Creator2/8  "xddot_WRL"
  Base Excitation/1 -> Bus Selector1/1
  Bus Selector1/1 -> Derivative/1, MATLAB Function19/42(y_FR)  "<y_FR>"
  Bus Selector1/2 -> Derivative1/1, MATLAB Function19/43(y_FL)  "<y_FL>"
  Bus Selector1/3 -> Derivative2/1, MATLAB Function19/44(y_RR)  "<y_RR>"
  Bus Selector1/4 -> Derivative3/1, MATLAB Function19/45(y_RL)  "<y_RL>"
  Derivative/1 -> MATLAB Function19/46(ydot_FR)
  Derivative1/1 -> MATLAB Function19/47(ydot_FL)
  Derivative2/1 -> MATLAB Function19/48(ydot_RR)
  Derivative3/1 -> MATLAB Function19/49(ydot_RL)
  Suspension Parameters/1 -> Bus Selector2/1
  Bus Selector2/1 -> MATLAB Function19/18(k_SFR)  "<k_SFR>"
  Bus Selector2/2 -> MATLAB Function19/19(k_SFL)  "<k_SFL>"
  Bus Selector2/3 -> MATLAB Function19/20(k_SRR)  "<k_SRR>"
  Bus Selector2/4 -> MATLAB Function19/21(k_SRL)  "<k_SRL>"
  Bus Selector2/9 -> MATLAB Function19/26(c_SFR)  "<c_SFR>"
  Bus Selector2/10 -> MATLAB Function19/27(c_SFL)  "<c_SFL>"
  Bus Selector2/11 -> MATLAB Function19/28(c_SRR)  "<c_SRR>"
  Bus Selector2/12 -> MATLAB Function19/29(c_SRL)  "<c_SRL>"
  Bus Selector2/5 -> MATLAB Function19/22(k_TFR)  "<k_TFR>"
  Bus Selector2/6 -> MATLAB Function19/23(k_TFL)  "<k_TFL>"
  Bus Selector2/7 -> MATLAB Function19/24(k_TRR)  "<k_TRR>"
  Bus Selector2/8 -> MATLAB Function19/25(k_TRL)  "<k_TRL>"
  Bus Selector2/13 -> MATLAB Function19/30(c_TFR)  "<c_TFR>"
  Bus Selector2/14 -> MATLAB Function19/31(c_TFL)  "<c_TFL>"
  Bus Selector2/15 -> MATLAB Function19/32(c_TRR)  "<c_TRR>"
  Bus Selector2/16 -> MATLAB Function19/33(c_TRL)  "<c_TRL>"
  Chassis Forces/1 -> Bus Selector3/1
  Bus Selector3/1 -> MATLAB Function19/34(F_zC)  "<F_z>"
  Bus Selector3/2 -> MATLAB Function19/35(M_y)  "<M_y>"
  Bus Selector3/3 -> MATLAB Function19/36(M_xF)  "<M_xF>"
  Bus Selector3/4 -> MATLAB Function19/37(M_xR)  "<M_xR>"
  Bus Selector4/1 -> MATLAB Function22/2(m_WFR)  "<m_WFR>"
  Bus Selector4/2 -> MATLAB Function22/3(m_WFL)  "<m_WFL>"
  Bus Selector4/3 -> MATLAB Function22/4(m_WRR)  "<m_WRR>"
  Bus Selector4/4 -> MATLAB Function22/5(m_WRL)  "<m_WRL>"
  Environment Parameters/1 -> Bus Selector5/1
  MATLAB Function22/1(F_zWFR) -> MATLAB Function19/38(F_zWFR)
  MATLAB Function22/2(F_zWFL) -> MATLAB Function19/39(F_zWFL)
  MATLAB Function22/3(F_zWRR) -> MATLAB Function19/40(F_zWRR)
  MATLAB Function22/4(F_zWRL) -> MATLAB Function19/41(F_zWRL)
  Bus Selector5/1 -> MATLAB Function22/1(g)  "<g>"

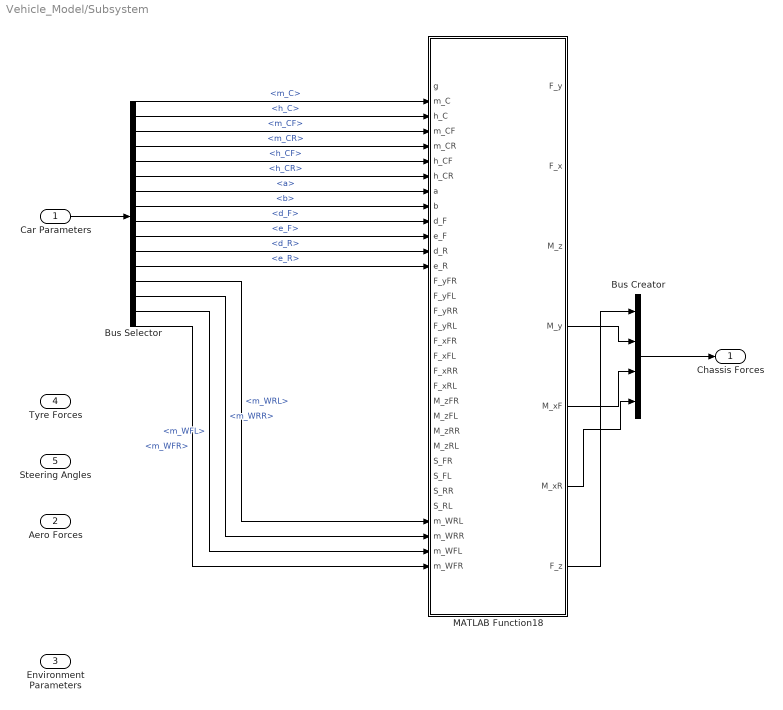
== system Vehicle_Model/Subsystem ==
  Car Parameters : Inport
  Aero Forces : Inport  Port=2
  Environment Parameters : Inport  Port=3
  Tyre Forces : Inport  Port=4
  Steering Angles : Inport  Port=5
  Bus Creator : BusCreator  Inputs=4
  Bus Selector : BusSelector  OutputSignals=m_C,h_C,m_CF,m_CR,h_CF,h_CR,a,b,d_F,e_F,d_R,e_R,m_WRL,m_WRR,m_WFL,m_WFR
  MATLAB Function18 : MATLAB Function  TreatAsAtomicUnit=on
  Chassis Forces : Outport
  wires:
  MATLAB Function18/7(F_z) -> Bus Creator/1
  MATLAB Function18/4(M_y) -> Bus Creator/2
  MATLAB Function18/5(M_xF) -> Bus Creator/3
  MATLAB Function18/6(M_xR) -> Bus Creator/4
  Bus Creator/1 -> Chassis Forces/1
  Car Parameters/1 -> Bus Selector/1
  Bus Selector/1 -> MATLAB Function18/2(m_C)  "<m_C>"
  Bus Selector/2 -> MATLAB Function18/3(h_C)  "<h_C>"
  Bus Selector/3 -> MATLAB Function18/4(m_CF)  "<m_CF>"
  Bus Selector/4 -> MATLAB Function18/5(m_CR)  "<m_CR>"
  Bus Selector/5 -> MATLAB Function18/6(h_CF)  "<h_CF>"
  Bus Selector/6 -> MATLAB Function18/7(h_CR)  "<h_CR>"
  Bus Selector/7 -> MATLAB Function18/8(a)  "<a>"
  Bus Selector/8 -> MATLAB Function18/9(b)  "<b>"
  Bus Selector/9 -> MATLAB Function18/10(d_F)  "<d_F>"
  Bus Selector/10 -> MATLAB Function18/11(e_F)  "<e_F>"
  Bus Selector/11 -> MATLAB Function18/12(d_R)  "<d_R>"
  Bus Selector/12 -> MATLAB Function18/13(e_R)  "<e_R>"
  Bus Selector/16 -> MATLAB Function18/33(m_WFR)  "<m_WFR>"
  Bus Selector/15 -> MATLAB Function18/32(m_WFL)  "<m_WFL>"
  Bus Selector/14 -> MATLAB Function18/31(m_WRR)  "<m_WRR>"
  Bus Selector/13 -> MATLAB Function18/30(m_WRL)  "<m_WRL>"

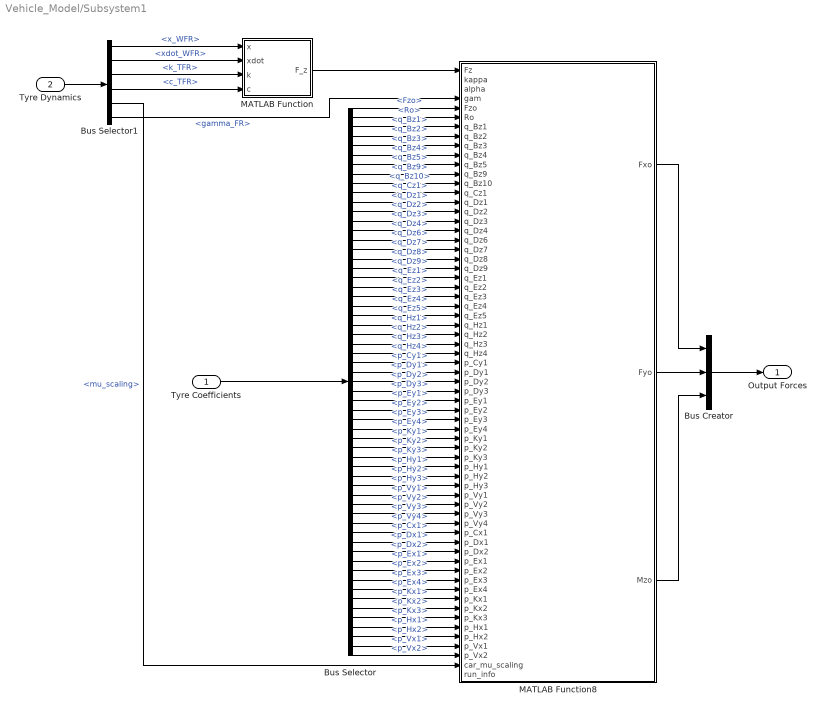
== system Vehicle_Model/Subsystem1 ==
  Tyre Coefficients : Inport
  Tyre Dynamics : Inport  Port=2
  Bus Creator : BusCreator  Inputs=3
  Bus Selector : BusSelector  OutputSignals=Fzo,Ro,q_Bz1,q_Bz2,q_Bz3,q_Bz4,q_Bz5,q_Bz9,q_Bz10,q_Cz1,q_Dz1,q_Dz2,q_Dz3,q_Dz4,q_Dz6,q_Dz7,q_Dz8,q_Dz9,q_Ez1,q_Ez2,q_Ez3,q_Ez4,q_Ez5,q_Hz1,q_Hz2,q_Hz3,q_Hz4,p_Cy1,p_Dy1,p_Dy2,p_Dy3,p_Ey1,p_Ey2,p_Ey3,p_Ey4,p_Ky1,p_Ky2,p_Ky3,p_Hy1,p_Hy2,p_Hy3,p_Vy1,p_Vy2,p_Vy3,p_Vy4,p_Cx1,p_Dx1,p_Dx2,p_Ex1,p_Ex2,p_Ex3,p_Ex4,p_Kx1,p_Kx2,p_Kx3,p_Hx1,p_Hx2,p_Vx1,p_Vx2
  Bus Selector1 : BusSelector  OutputSignals=x_WFR,xdot_WFR,signal3.k_TFR,signal3.c_TFR,mu_scaling,signal3.gamma_FR
  MATLAB Function : MATLAB Function  TreatAsAtomicUnit=on
  MATLAB Function8 : MATLAB Function  TreatAsAtomicUnit=on
  Output Forces : Outport
  wires:
  MATLAB Function8/2(Fyo) -> Bus Creator/2
  MATLAB Function8/1(Fxo) -> Bus Creator/1
  MATLAB Function8/3(Mzo) -> Bus Creator/3
  Bus Creator/1 -> Output Forces/1
  Tyre Coefficients/1 -> Bus Selector/1
  Bus Selector/1 -> MATLAB Function8/5(Fzo)  "<Fzo>"
  Bus Selector/2 -> MATLAB Function8/6(Ro)  "<Ro>"
  Bus Selector/3 -> MATLAB Function8/7(q_Bz1)  "<q_Bz1>"
  Bus Selector/4 -> MATLAB Function8/8(q_Bz2)  "<q_Bz2>"
  Bus Selector/5 -> MATLAB Function8/9(q_Bz3)  "<q_Bz3>"
  Bus Selector/6 -> MATLAB Function8/10(q_Bz4)  "<q_Bz4>"
  Bus Selector/7 -> MATLAB Function8/11(q_Bz5)  "<q_Bz5>"
  Bus Selector/8 -> MATLAB Function8/12(q_Bz9)  "<q_Bz9>"
  Bus Selector/9 -> MATLAB Function8/13(q_Bz10)  "<q_Bz10>"
  Bus Selector/10 -> MATLAB Function8/14(q_Cz1)  "<q_Cz1>"
  Bus Selector/11 -> MATLAB Function8/15(q_Dz1)  "<q_Dz1>"
  Bus Selector/12 -> MATLAB Function8/16(q_Dz2)  "<q_Dz2>"
  Bus Selector/13 -> MATLAB Function8/17(q_Dz3)  "<q_Dz3>"
  Bus Selector/14 -> MATLAB Function8/18(q_Dz4)  "<q_Dz4>"
  Bus Selector/15 -> MATLAB Function8/19(q_Dz6)  "<q_Dz6>"
  Bus Selector/16 -> MATLAB Function8/20(q_Dz7)  "<q_Dz7>"
  Bus Selector/17 -> MATLAB Function8/21(q_Dz8)  "<q_Dz8>"
  Bus Selector/18 -> MATLAB Function8/22(q_Dz9)  "<q_Dz9>"
  Bus Selector/19 -> MATLAB Function8/23(q_Ez1)  "<q_Ez1>"
  Bus Selector/20 -> MATLAB Function8/24(q_Ez2)  "<q_Ez2>"
  Bus Selector/21 -> MATLAB Function8/25(q_Ez3)  "<q_Ez3>"
  Bus Selector/22 -> MATLAB Function8/26(q_Ez4)  "<q_Ez4>"
  Bus Selector/23 -> MATLAB Function8/27(q_Ez5)  "<q_Ez5>"
  Bus Selector/24 -> MATLAB Function8/28(q_Hz1)  "<q_Hz1>"
  Bus Selector/25 -> MATLAB Function8/29(q_Hz2)  "<q_Hz2>"
  Bus Selector/26 -> MATLAB Function8/30(q_Hz3)  "<q_Hz3>"
  Bus Selector/27 -> MATLAB Function8/31(q_Hz4)  "<q_Hz4>"
  Bus Selector/28 -> MATLAB Function8/32(p_Cy1)  "<p_Cy1>"
  Bus Selector/29 -> MATLAB Function8/33(p_Dy1)  "<p_Dy1>"
  Bus Selector/30 -> MATLAB Function8/34(p_Dy2)  "<p_Dy2>"
  Bus Selector/31 -> MATLAB Function8/35(p_Dy3)  "<p_Dy3>"
  Bus Selector/32 -> MATLAB Function8/36(p_Ey1)  "<p_Ey1>"
  Bus Selector/33 -> MATLAB Function8/37(p_Ey2)  "<p_Ey2>"
  Bus Selector/34 -> MATLAB Function8/38(p_Ey3)  "<p_Ey3>"
  Bus Selector/35 -> MATLAB Function8/39(p_Ey4)  "<p_Ey4>"
  Bus Selector/36 -> MATLAB Function8/40(p_Ky1)  "<p_Ky1>"
  Bus Selector/37 -> MATLAB Function8/41(p_Ky2)  "<p_Ky2>"
  Bus Selector/38 -> MATLAB Function8/42(p_Ky3)  "<p_Ky3>"
  Bus Selector/39 -> MATLAB Function8/43(p_Hy1)  "<p_Hy1>"
  Bus Selector/40 -> MATLAB Function8/44(p_Hy2)  "<p_Hy2>"
  Bus Selector/41 -> MATLAB Function8/45(p_Hy3)  "<p_Hy3>"
  Bus Selector/42 -> MATLAB Function8/46(p_Vy1)  "<p_Vy1>"
  Bus Selector/43 -> MATLAB Function8/47(p_Vy2)  "<p_Vy2>"
  Bus Selector/44 -> MATLAB Function8/48(p_Vy3)  "<p_Vy3>"
  Bus Selector/45 -> MATLAB Function8/49(p_Vy4)  "<p_Vy4>"
  Bus Selector/46 -> MATLAB Function8/50(p_Cx1)  "<p_Cx1>"
  Bus Selector/47 -> MATLAB Function8/51(p_Dx1)  "<p_Dx1>"
  Bus Selector/48 -> MATLAB Function8/52(p_Dx2)  "<p_Dx2>"
  Bus Selector/49 -> MATLAB Function8/53(p_Ex1)  "<p_Ex1>"
  Bus Selector/50 -> MATLAB Function8/54(p_Ex2)  "<p_Ex2>"
  Bus Selector/51 -> MATLAB Function8/55(p_Ex3)  "<p_Ex3>"
  Bus Selector/52 -> MATLAB Function8/56(p_Ex4)  "<p_Ex4>"
  Bus Selector/53 -> MATLAB Function8/57(p_Kx1)  "<p_Kx1>"
  Bus Selector/54 -> MATLAB Function8/58(p_Kx2)  "<p_Kx2>"
  Bus Selector/55 -> MATLAB Function8/59(p_Kx3)  "<p_Kx3>"
  Bus Selector/56 -> MATLAB Function8/60(p_Hx1)  "<p_Hx1>"
  Bus Selector/57 -> MATLAB Function8/61(p_Hx2)  "<p_Hx2>"
  Bus Selector/58 -> MATLAB Function8/62(p_Vx1)  "<p_Vx1>"
  Bus Selector/59 -> MATLAB Function8/63(p_Vx2)  "<p_Vx2>"
  Tyre Dynamics/1 -> Bus Selector1/1
  Bus Selector1/1 -> MATLAB Function/1(x)  "<x_WFR>"
  Bus Selector1/2 -> MATLAB Function/2(xdot)  "<xdot_WFR>"
  MATLAB Function/1(F_z) -> MATLAB Function8/1(Fz)
  Bus Selector1/3 -> MATLAB Function/3(k)  "<k_TFR>"
  Bus Selector1/4 -> MATLAB Function/4(c)  "<c_TFR>"
  Bus Selector1/5 -> MATLAB Function8/64(car_mu_scaling)  "<mu_scaling>"
  Bus Selector1/6 -> MATLAB Function8/4(gam)  "<gamma_FR>"

== matlab function Vehicle_Model/MATLAB Function1 ==
  data: m_C output; m_CF output; m_CR output; m_WFR output; m_WFL output; m_WRR output; m_WRL output; I_Cy output; I_CFx output; I_CRx output; a output; b output; d_F output; e_F output; d_R output; e_R output; k_SFR output; k_SFL output; k_SRR output; k_SRL output; k_TFR output; k_TFL output; k_TRR output; k_TRL output; c_SFR output; c_SFL output; c_SRR output; c_SRL output; c_TFR output; c_TFL output; c_TRR output; c_TRL output; k_C output; c_C output; h_C output; h_CF output; h_CR output
function [m_C,m_CF,m_CR,m_WFR,m_WFL,m_WRR,m_WRL,I_Cy,I_CFx,I_CRx,a,b,d_F,e_F,d_R,e_R,...
    k_SFR,k_SFL,k_SRR,k_SRL,k_TFR,k_TFL,k_TRR,k_TRL,c_SFR,c_SFL,c_SRR,c_SRL,...
    c_TFR,c_TFL,c_TRR,c_TRL,k_C,c_C,h_C,h_CF,h_CR] = Car_Parameters
%% Car Parameters
% Masses
m_C = 200; %car sprung mass (kg)
m_CF = 100;
m_CR = m_C - m_CF;
m_WFR = 5; %front right wheel mass (kg)
m_WFL = 5; %front left wheel mass (kg)
m_WRR = 5; %rear right wheel mass (kg)
m_WRL = 5; %rear left wheel mass (kg)

% Intertias
I_Cy = 1000; %chassis interia around y (kg m^2)
I_CFx = 500; %chassis front inertia around x (kg m^2)
I_CRx = 500; %chassis rear inertia around x (kg m^2)

% Geometries
a = 0.8; %distance of COG from front axle (m)
b = 0.8; %distance of COG from rear axle (m)
d_F = 0.6; %distance of COG from front left tire (m)
e_F = 0.6; %distance of COG from front right tire (m)
d_R = 0.6; %distance of COG from rear left tire (m)
e_R = 0.6; %distance of COG from rear right tire (m)
h_C = 0.4;
h_CF = 0.4;
h_CR = 0.4;

% Suspension Stifnesses
k_SFR = 2000; %suspension stiffness front right (N/m)
k_SFL = 2000; %suspension stiffness front left (N/m)
k_SRR = 2000; %suspension stiffness rear right (N/m)
k_SRL = 2000; %suspension stiffness rear left (N/m)

% Tire Stifnesses
k_TFR = 15000; %tire stiffness front right (N/m)
k_TFL = 15000; %tire stiffness front left (N/m)
k_TRR = 15000; %tire stiffness rear right (N/m)
k_TRL = 15000; %tire stiffness rear left (N/m)

% Suspension Damping Coefficients
c_SFR = 1000; %suspension damping coefficient front right (Ns/m)
c_SFL = 1000; %suspension damping coefficient front left (Ns/m)
c_SRR = 1000; %suspension damping coefficientv rear right (Ns/m)
c_SRL = 1000; %suspension damping coefficient rear left (Ns/m)

% Tire Damping Coefficients
c_TFR = 500; %tire damping coefficient front right (Ns/m)
c_TFL = 500; %tire damping coefficient front left (Ns/m)
c_TRR = 500; %tire damping coefficientv rear right (Ns/m)
c_TRL = 500; %tire damping coefficient rear left (Ns/m)

% Other Stiffnesses
k_C = 2000;

% Other Damping Coefficients
c_C = 1000;
